simulink model "pendulo"  (R2025a)
settings: Solver=VariableStepAuto  StartTime=0.0  StopTime=1000.0  RelTol=1e-3
values from neighbouring files (symbols this model uses):
  a_init = 0.0174532925199    [matlab.mat]
  Beq = 4.3    [matlab.mat]
  Bp = 0.0024    [matlab.mat]
  Fc = 0    [matlab.mat]
  g = 9.81    [matlab.mat]
  Ip = 79    [matlab.mat]
  Lp = 0.3302    [matlab.mat]
  Mc = 0.23    [matlab.mat]
  Mp = 0.23    [matlab.mat]
settings Model: Creator=joshi  LastModifiedBy=joshi

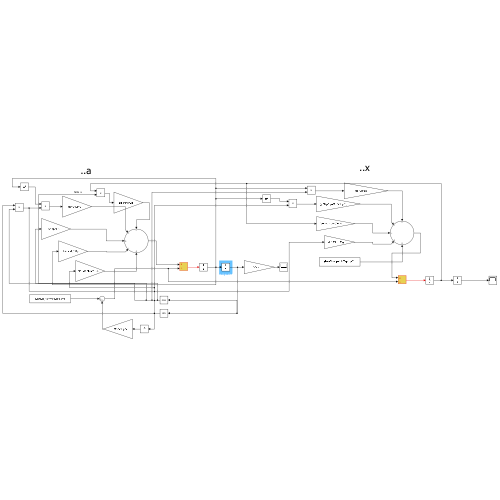
[thumbnail: Simulink's stored preview of the top-level diagram]
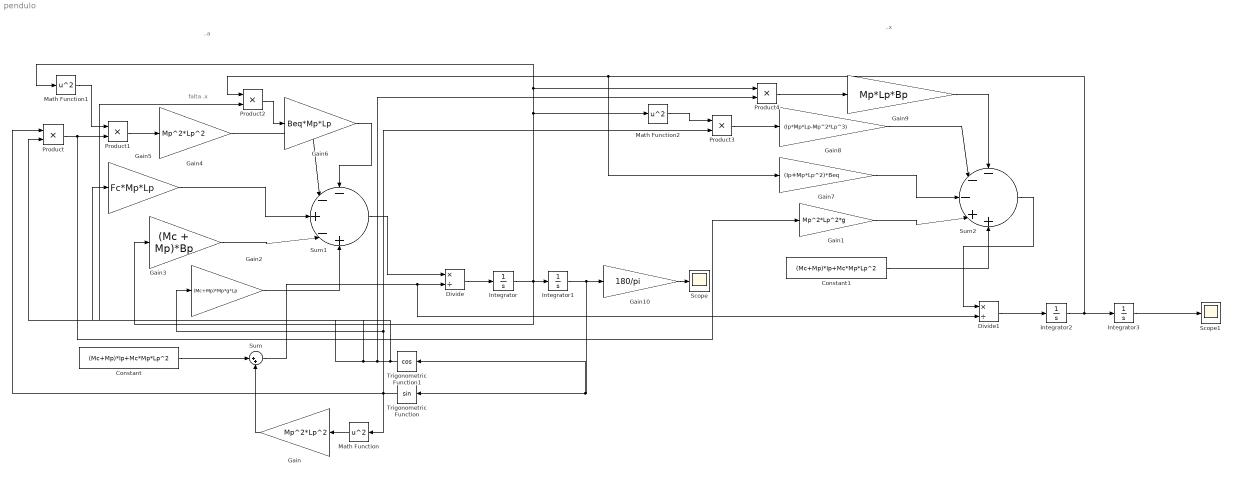
== system pendulo ==
  note: ..a
  note: falta .x
  note: ..x
  Constant : Constant  Value=(Mc+Mp)*Ip+Mc*Mp*Lp^2
  Constant1 : Constant  Value=(Mc+Mp)*Ip+Mc*Mp*Lp^2
  Divide : Product  Inputs=*/
  Divide1 : Product  Inputs=*/
  Gain : Gain  Gain=Mp^2*Lp^2
  Gain1 : Gain  Gain=Mp^2*Lp^2*g
  Gain10 : Gain  Gain=180/pi
  Gain2 : Gain  Gain=(Mc+Mp)*Mp*g*Lp
  Gain3 : Gain  Gain=(Mc + Mp)*Bp
  Gain4 : Gain  Gain=Mp^2*Lp^2
  Gain5 : Gain  Gain=Fc*Mp*Lp
  Gain6 : Gain  Gain=Beq*Mp*Lp
  Gain7 : Gain  Gain=(Ip+Mp*Lp^2)*Beq
  Gain8 : Gain  Gain=(Ip*Mp*Lp-Mp^2*Lp^3)
  Gain9 : Gain  Gain=Mp*Lp*Bp
  Integrator : Integrator
  Integrator1 : Integrator  InitialCondition=a_init
  Integrator2 : Integrator
  Integrator3 : Integrator
  Math Function : Math  Operator=square
  Math Function1 : Math  Operator=square
  Math Function2 : Math  Operator=square
  Product{,1..4} (5 alike) : Product
  Scope : Scope
      settings: Title=Alpha  ActiveDisplayYMinimum=-391.49008977218551  ActiveDisplayYMaximum=44.610012388945627
  Scope1 : Scope
      settings: Title=X  ActiveDisplayYMinimum=-13.369826163559271  ActiveDisplayYMaximum=120.32843547203348
  Sum : Sum  Inputs=|++
  Sum1 : Sum  Inputs=--+-+
  Sum2 : Sum  Inputs=---++
  Trigonometric Function : Trigonometry
  Trigonometric Function1 : Trigonometry  Operator=cos
  wires:
  Integrator/1 -> Math Function2/1, Product4/1, Math Function1/1, Gain3/1, Integrator1/1
  Integrator1/1 -> Gain10/1, Trigonometric Function1/1, Trigonometric Function/1
  Trigonometric Function/1 -> Product3/2, Gain2/1, Product/1, Math Function/1
  Math Function/1 -> Gain/1
  Gain/1 -> Sum/2
  Sum/1 -> Divide1/2, Divide/2
  Divide/1 -> Integrator/1
  Sum1/1 -> Divide/1
  Gain2/1 -> Sum1/5
  Gain3/1 -> Sum1/4
  Product/1 -> Gain1/1, Product1/2
  Trigonometric Function1/1 -> Gain5/1, Product2/2, Product/2, Product4/2
  Math Function1/1 -> Product1/1
  Product1/1 -> Gain4/1
  Gain4/1 -> Sum1/2
  Gain5/1 -> Sum1/3
  Gain6/1 -> Sum1/1
  Product2/1 -> Gain6/1
  Sum2/1 -> Divide1/1
  Constant/1 -> Sum/1
  Divide1/1 -> Integrator2/1
  Integrator2/1 -> Gain7/1, Product2/1, Integrator3/1
  Constant1/1 -> Sum2/5
  Gain1/1 -> Sum2/4
  Integrator3/1 -> Scope1/1
  Gain7/1 -> Sum2/3
  Gain8/1 -> Sum2/2
  Product3/1 -> Gain8/1
  Math Function2/1 -> Product3/1
  Product4/1 -> Gain9/1
  Gain9/1 -> Sum2/1
  Gain10/1 -> Scope/1
